simulink model "M_M_m_K_N"  (R2024b)
settings: Solver=VariableStepAuto  StartTime=0.0  StopTime=50000  RelTol=1e-3
values from neighbouring files (symbols this model uses):
  m = 1    [MMmKN_indicatori.m]    (also in MMmK_indicatori.m = 2; Perf_M_M_m.m = m(:)'; Perf_M_M_m_K.m = m(:)'; Perf_M_M_m_K_N.m = m(:)')
undefined symbols (not defined in the file or in its folder): n
settings Model: Creator=uig58269  LastModifiedBy=atomu
settings RTWCC: GPUComputeCapability=3.5

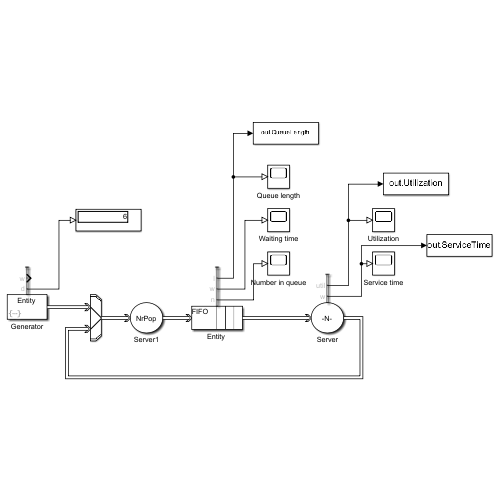
[thumbnail: Simulink's stored preview of the top-level diagram]
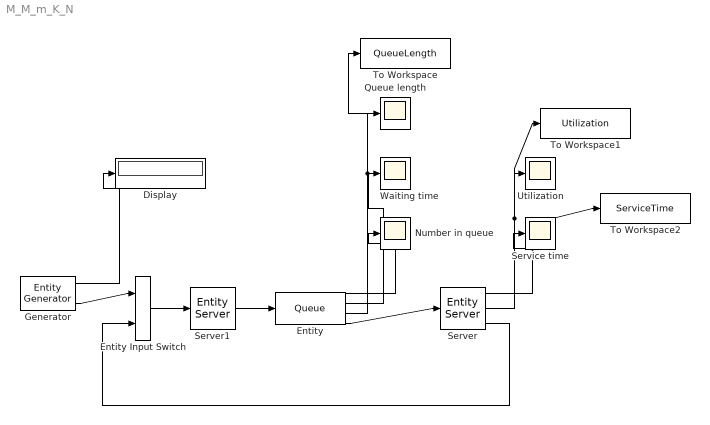
== system M_M_m_K_N ==
  Display : Display
  Entity Input Switch : EntityInputSwitch  InputPortMessageModes=m,m  OutputPortMessageModes=m
  "Entity " : Queue  InputPortMessageModes=m  OutputPortMessageModes=n,n,n,m  Capacity=MaxReq - ServerNumbers  NumberEntitiesInBlock=on  AverageWait=on  AverageQueueLength=on
      settings: OutputPortMap=o1,o2,o3,o5
  Generator : EntityGenerator  OutputPortMessageModes=n,n,m  TimeSource=MATLAB action  IntergenerationTimeAction=|  GenerateEntityAtSimulationStart=off  GenerateAction=|  AttributeName=TimeStamp  AttributeInitialValue=0  NumberEntitiesDeparted=on  AverageIntergenerationTime=on  EntityType=Structured  EntityTypeName=Entity
      IntergenerationTimeAction=|
      | persistent rngInit;
      | if isempty(rngInit)
      |     seed = 12345;
      |     rng(seed);
      |     rngInit = true;
      | end
      | 
      | % Pattern: Repeating Sequence
      | persistent SEQ;
      | persistent idx;
      | if isempty(SEQ)
      |     SEQ = [zeros(1,NrPop) inf];
      |     idx = 1;
      | end
      | if idx > numel(SEQ)
      |     idx = 1;
      | end
      | dt = SEQ(idx);
      | idx = idx + 1;
      GenerateAction=|
      | % Record time of generation so we can
      | % compute system time
      settings: OutputPortMap=o0,o2,o3
  Number in queue : Scope
  Queue length : Scope
  Server : EntityServer  InputPortMessageModes=m  OutputPortMessageModes=n,n,m  Capacity=ServerNumbers  ServiceTimeSource=MATLAB action  ServiceTimeAction=|  AverageWait=on  Utilization=on
      | persistent rngInit;
      | if isempty(rngInit)
      |     seed = 93521;
      |     rng(seed);
      |     rngInit = true;
      | end
      | 
      | % Pattern: Exponential distribution
      | med= 1/mu;
      | dt = -med * log(1 - rand());
      settings: OutputPortMap=o4,o5,o9
  Server1 : EntityServer  InputPortMessageModes=m  OutputPortMessageModes=m  Capacity=NrPop  ServiceTimeSource=MATLAB action  ServiceTimeAction=|
      | persistent rngInit;
      | if isempty(rngInit)
      |     seed = 25487;
      |     rng(seed);
      |     rngInit = true;
      | end
      | 
      | % Pattern: Exponential distribution
      | mu= 1/lambda;
      | dt = -mu * log(1 - rand());
  Service time : Scope
  To Workspace : ToWorkspace  VariableName=QueueLength  SaveFormat=Timeseries  SampleTime=-1
  To Workspace1 : ToWorkspace  VariableName=Utilization  SaveFormat=Timeseries  SampleTime=-1
  To Workspace2 : ToWorkspace  VariableName=ServiceTime  SaveFormat=Timeseries  SampleTime=-1
  Utilization : Scope
  Waiting time : Scope
  wires:
  "Entity "/2 -> Waiting time/1
  Server/3 -> Entity Input Switch/2
  Server/1 -> To Workspace2/1, Service time/1
  "Entity "/3 -> To Workspace/1, Queue length/1
  "Entity "/4 -> Server/1
  Server/2 -> To Workspace1/1, Utilization/1
  "Entity "/1 -> Number in queue/1
  Entity Input Switch/1 -> Server1/1
  Server1/1 -> "Entity "/1
  Generator/3 -> Entity Input Switch/1
  Generator/1 -> Display/1
